simulink model "Motors_PID_Simulink_Cosimulation"  (R2019b)
settings: Solver=VariableStepAuto  StartTime=0.0  StopTime=10  FixedStep=0.0001  RelTol=1e-3
values from neighbouring files (symbols this model uses):
  desired_angle_vectors = deg2rad(desired_angles_deg)    [Motors_Main_Project.m]
  EKb = Kb(3)    [Motors_Main_Project.m]
  EKm = Km(3)    [Motors_Main_Project.m]
  EL = L(3)    [Motors_Main_Project.m]
  SKb = Kb(4)    [Motors_Main_Project.m]
  SKm = Km(4)    [Motors_Main_Project.m]
  SL = L(4)    [Motors_Main_Project.m]
  WKb = Kb(2)    [Motors_Main_Project.m]
  WKm = Km(2)    [Motors_Main_Project.m]
  WL = L(2)    [Motors_Main_Project.m]
undefined symbols (not defined in the file or in its folder): ER, GR, SR
libraries: cstblocks x4, simulink x4
settings Model: Creator=harsh  LastModifiedBy=harsh

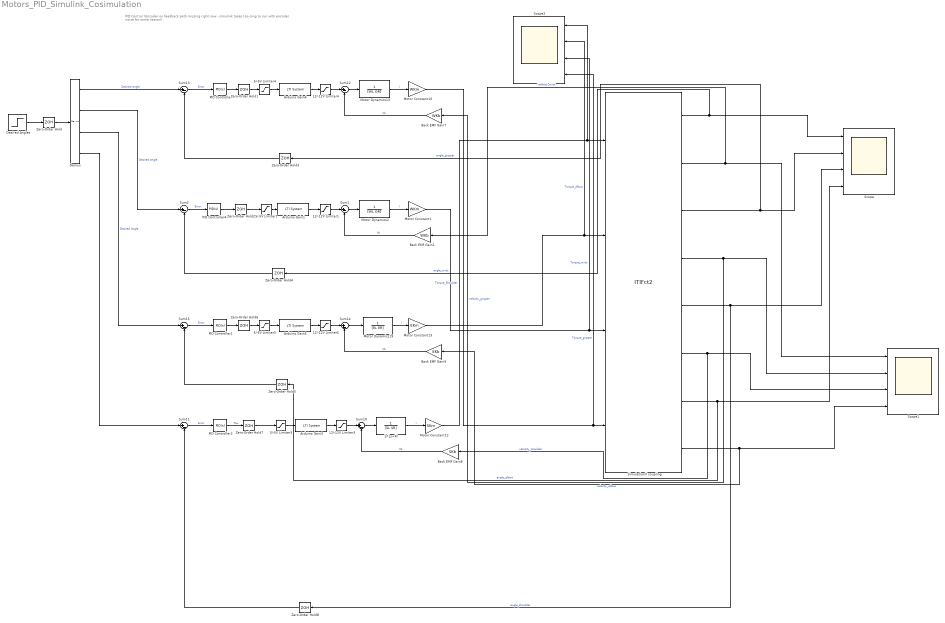
== system Motors_PID_Simulink_Cosimulation ==
  note: PID Control
      | (Encoder on feedback path missing right now - simulink takes too long to run with encoder noise for some reason)
  1/(Ls+R) : TransferFcn  Denominator=[SL SR]
  12/-12V Limiter{1,3..5} (4 alike) : Saturate  UpperLimit=12  LowerLimit=-12
  5/-5V Limiter{1,3..5} (4 alike) : Saturate  UpperLimit=5  LowerLimit=-5
  Arduino Gain1 : cstblocks/LTI System  sys=WOPAMP  IC=[]
  Arduino Gain3 : cstblocks/LTI System  sys=SOPAMP  IC=[]
  Arduino Gain4 : cstblocks/LTI System  sys=GOPAMP  IC=[]
  Arduino Gain5 : cstblocks/LTI System  sys=EOPAMP  IC=[]
  Back EMF Gain1 : Gain  Gain=WKb
  Back EMF Gain7 : Gain  Gain=WKb
  Back EMF Gain8 : Gain  Gain=SKb
  Back EMF Gain9 : Gain  Gain=EKb
  Demux : Demux
  "Desired Angles " : Step  Time=0.1  After=desired_angle_vectors  SampleTime=0
  Motor Constant1 : Gain  Gain=WKm
  Motor Constant10 : Gain  Gain=WKm
  Motor Constant12 : Gain  Gain=SKm
  Motor Constant13 : Gain  Gain=EKm
  Motor Dynamics13 : TransferFcn  Denominator=[WL GR]
  Motor Dynamics19 : TransferFcn  Denominator=[EL ER]
  Motor Dynamics2 : TransferFcn  Denominator=[WL GR]
  PID Controller : simulink/Continuous/PID Controller  Controller=PID  Form=Parallel  TimeDomain=Continuous-time  SampleTime=-1  IntegratorMethod=Forward Euler  FilterMethod=Forward Euler  ControllerParametersSource=internal  P=0.3697  I=0.00525  D=0.54744  UseFilter=on  N=5000  TunerSelectOption=Transfer Function Based (PID Tuner App)  InitialConditionSource=internal  InitialConditionForIntegrator=0  InitialConditionForFilter=0  DifferentiatorICPrevScaledInput=0  ExternalReset=none  TrackingMode=off  Kt=1  LimitOutput=off  UpperSaturationLimit=inf  LowerSaturationLimit=-inf  LinearizeAsGain=on  AntiWindupMode=none  Kb=1  POutMin=[]  POutMax=[]  IOutMin=[]  IOutMax=[]  DOutMin=[]  DOutMax=[]  NOutMin=[]  NOutMax=[]  SumOutMin=[]  SumOutMax=[]  SaturationOutMin=[]  SaturationOutMax=[]  PParamMin=[]  PParamMax=[]  IParamMin=[]  IParamMax=[]  DParamMin=[]  DParamMax=[]  NParamMin=[]  NParamMax=[]  KbParamMin=[]  KbParamMax=[]  KtParamMin=[]  KtParamMax=[]  KbOutMin=[]  KbOutMax=[]  KtOutMin=[]  KtOutMax=[]  IntegratorOutMin=[]  IntegratorOutMax=[]  FilterOutMin=[]  FilterOutMax=[]  SumI1OutMin=[]  SumI1OutMax=[]  SumI2OutMin=[]  SumI2OutMax=[]  SumI3OutMin=[]  SumI3OutMax=[]  SumI4OutMin=[]  SumI4OutMax=[]  SumDOutMin=[]  SumDOutMax=[]  DifferentiatorOutMin=[]  DifferentiatorOutMax=[]  FilterDiffOutCoefMin=[]  FilterDiffOutCoefMax=[]  ReciprocalOutMin=[]  ReciprocalOutMax=[]  SumDenOutMin=[]  SumDenOutMax=[]  SumNumOutMin=[]  SumNumOutMax=[]  DivideOutMin=[]  DivideOutMax=[]  IntegratorContinuousStateAttributes=''  IntegratorStateMustResolveToSignalObject=off  IntegratorRTWStateStorageClass=Auto  FilterContinuousStateAttributes=''  FilterStateMustResolveToSignalObject=off  FilterRTWStateStorageClass=Auto  ParallelPVariant=InternalParameters  IdealPVariant=Disabled  IVariant=InternalParameters  DVariant=InternalParameters  IntegratorVariant=Continuous  SatVariant=Disabled  AWVariant=Passthrough  PCopyVariant=Disabled  TRVariant=Disabled  FdbkBlocksVariant=Forward  IdealPFdbkVariant=Disabled  SatFdbkVariant=Disabled  DerivativeFilterVariant=ContFilter  NVariant=InternalParameters  NCopyVariant=Disabled  FilterICVariant=InternalICsFilter  IntegratorICVariant=InternalICs  ExternalResetVariant=Disabled  TRSumVariant=Passthrough  SumFdbkVariant=Disabled  SumVariant=Sum_PID
  PID Controller1 : simulink/Continuous/PID Controller  Controller=PID  Form=Parallel  TimeDomain=Continuous-time  SampleTime=-1  IntegratorMethod=Forward Euler  FilterMethod=Forward Euler  ControllerParametersSource=internal  P=0.03697  I=0.000525  D=3.84744  UseFilter=on  N=5000  TunerSelectOption=Transfer Function Based (PID Tuner App)  InitialConditionSource=internal  InitialConditionForIntegrator=0  InitialConditionForFilter=0  DifferentiatorICPrevScaledInput=0  ExternalReset=none  TrackingMode=off  Kt=1  LimitOutput=off  UpperSaturationLimit=inf  LowerSaturationLimit=-inf  LinearizeAsGain=on  AntiWindupMode=none  Kb=1  POutMin=[]  POutMax=[]  IOutMin=[]  IOutMax=[]  DOutMin=[]  DOutMax=[]  NOutMin=[]  NOutMax=[]  SumOutMin=[]  SumOutMax=[]  SaturationOutMin=[]  SaturationOutMax=[]  PParamMin=[]  PParamMax=[]  IParamMin=[]  IParamMax=[]  DParamMin=[]  DParamMax=[]  NParamMin=[]  NParamMax=[]  KbParamMin=[]  KbParamMax=[]  KtParamMin=[]  KtParamMax=[]  KbOutMin=[]  KbOutMax=[]  KtOutMin=[]  KtOutMax=[]  IntegratorOutMin=[]  IntegratorOutMax=[]  FilterOutMin=[]  FilterOutMax=[]  SumI1OutMin=[]  SumI1OutMax=[]  SumI2OutMin=[]  SumI2OutMax=[]  SumI3OutMin=[]  SumI3OutMax=[]  SumI4OutMin=[]  SumI4OutMax=[]  SumDOutMin=[]  SumDOutMax=[]  DifferentiatorOutMin=[]  DifferentiatorOutMax=[]  FilterDiffOutCoefMin=[]  FilterDiffOutCoefMax=[]  ReciprocalOutMin=[]  ReciprocalOutMax=[]  SumDenOutMin=[]  SumDenOutMax=[]  SumNumOutMin=[]  SumNumOutMax=[]  DivideOutMin=[]  DivideOutMax=[]  IntegratorContinuousStateAttributes=''  IntegratorStateMustResolveToSignalObject=off  IntegratorRTWStateStorageClass=Auto  FilterContinuousStateAttributes=''  FilterStateMustResolveToSignalObject=off  FilterRTWStateStorageClass=Auto  ParallelPVariant=InternalParameters  IdealPVariant=Disabled  IVariant=InternalParameters  DVariant=InternalParameters  IntegratorVariant=Continuous  SatVariant=Disabled  AWVariant=Passthrough  PCopyVariant=Disabled  TRVariant=Disabled  FdbkBlocksVariant=Forward  IdealPFdbkVariant=Disabled  SatFdbkVariant=Disabled  DerivativeFilterVariant=ContFilter  NVariant=InternalParameters  NCopyVariant=Disabled  FilterICVariant=InternalICsFilter  IntegratorICVariant=InternalICs  ExternalResetVariant=Disabled  TRSumVariant=Passthrough  SumFdbkVariant=Disabled  SumVariant=Sum_PID
  PID Controller2 : simulink/Continuous/PID Controller  Controller=PID  Form=Parallel  TimeDomain=Continuous-time  SampleTime=-1  IntegratorMethod=Forward Euler  FilterMethod=Forward Euler  ControllerParametersSource=internal  P=0.03697  I=0.00525  D=0.84744  UseFilter=on  N=5000  TunerSelectOption=Transfer Function Based (PID Tuner App)  InitialConditionSource=internal  InitialConditionForIntegrator=0  InitialConditionForFilter=0  DifferentiatorICPrevScaledInput=0  ExternalReset=none  TrackingMode=off  Kt=1  LimitOutput=off  UpperSaturationLimit=inf  LowerSaturationLimit=-inf  LinearizeAsGain=on  AntiWindupMode=none  Kb=1  POutMin=[]  POutMax=[]  IOutMin=[]  IOutMax=[]  DOutMin=[]  DOutMax=[]  NOutMin=[]  NOutMax=[]  SumOutMin=[]  SumOutMax=[]  SaturationOutMin=[]  SaturationOutMax=[]  PParamMin=[]  PParamMax=[]  IParamMin=[]  IParamMax=[]  DParamMin=[]  DParamMax=[]  NParamMin=[]  NParamMax=[]  KbParamMin=[]  KbParamMax=[]  KtParamMin=[]  KtParamMax=[]  KbOutMin=[]  KbOutMax=[]  KtOutMin=[]  KtOutMax=[]  IntegratorOutMin=[]  IntegratorOutMax=[]  FilterOutMin=[]  FilterOutMax=[]  SumI1OutMin=[]  SumI1OutMax=[]  SumI2OutMin=[]  SumI2OutMax=[]  SumI3OutMin=[]  SumI3OutMax=[]  SumI4OutMin=[]  SumI4OutMax=[]  SumDOutMin=[]  SumDOutMax=[]  DifferentiatorOutMin=[]  DifferentiatorOutMax=[]  FilterDiffOutCoefMin=[]  FilterDiffOutCoefMax=[]  ReciprocalOutMin=[]  ReciprocalOutMax=[]  SumDenOutMin=[]  SumDenOutMax=[]  SumNumOutMin=[]  SumNumOutMax=[]  DivideOutMin=[]  DivideOutMax=[]  IntegratorContinuousStateAttributes=''  IntegratorStateMustResolveToSignalObject=off  IntegratorRTWStateStorageClass=Auto  FilterContinuousStateAttributes=''  FilterStateMustResolveToSignalObject=off  FilterRTWStateStorageClass=Auto  ParallelPVariant=InternalParameters  IdealPVariant=Disabled  IVariant=InternalParameters  DVariant=InternalParameters  IntegratorVariant=Continuous  SatVariant=Disabled  AWVariant=Passthrough  PCopyVariant=Disabled  TRVariant=Disabled  FdbkBlocksVariant=Forward  IdealPFdbkVariant=Disabled  SatFdbkVariant=Disabled  DerivativeFilterVariant=ContFilter  NVariant=InternalParameters  NCopyVariant=Disabled  FilterICVariant=InternalICsFilter  IntegratorICVariant=InternalICs  ExternalResetVariant=Disabled  TRSumVariant=Passthrough  SumFdbkVariant=Disabled  SumVariant=Sum_PID
  PID Controller4 : simulink/Continuous/PID Controller  Controller=PID  Form=Parallel  TimeDomain=Continuous-time  SampleTime=-1  IntegratorMethod=Forward Euler  FilterMethod=Forward Euler  ControllerParametersSource=internal  P=0.3697  I=0.00525  D=0.74744  UseFilter=on  N=5000  TunerSelectOption=Transfer Function Based (PID Tuner App)  InitialConditionSource=internal  InitialConditionForIntegrator=0  InitialConditionForFilter=0  DifferentiatorICPrevScaledInput=0  ExternalReset=none  TrackingMode=off  Kt=1  LimitOutput=off  UpperSaturationLimit=inf  LowerSaturationLimit=-inf  LinearizeAsGain=on  AntiWindupMode=none  Kb=1  POutMin=[]  POutMax=[]  IOutMin=[]  IOutMax=[]  DOutMin=[]  DOutMax=[]  NOutMin=[]  NOutMax=[]  SumOutMin=[]  SumOutMax=[]  SaturationOutMin=[]  SaturationOutMax=[]  PParamMin=[]  PParamMax=[]  IParamMin=[]  IParamMax=[]  DParamMin=[]  DParamMax=[]  NParamMin=[]  NParamMax=[]  KbParamMin=[]  KbParamMax=[]  KtParamMin=[]  KtParamMax=[]  KbOutMin=[]  KbOutMax=[]  KtOutMin=[]  KtOutMax=[]  IntegratorOutMin=[]  IntegratorOutMax=[]  FilterOutMin=[]  FilterOutMax=[]  SumI1OutMin=[]  SumI1OutMax=[]  SumI2OutMin=[]  SumI2OutMax=[]  SumI3OutMin=[]  SumI3OutMax=[]  SumI4OutMin=[]  SumI4OutMax=[]  SumDOutMin=[]  SumDOutMax=[]  DifferentiatorOutMin=[]  DifferentiatorOutMax=[]  FilterDiffOutCoefMin=[]  FilterDiffOutCoefMax=[]  ReciprocalOutMin=[]  ReciprocalOutMax=[]  SumDenOutMin=[]  SumDenOutMax=[]  SumNumOutMin=[]  SumNumOutMax=[]  DivideOutMin=[]  DivideOutMax=[]  IntegratorContinuousStateAttributes=''  IntegratorStateMustResolveToSignalObject=off  IntegratorRTWStateStorageClass=Auto  FilterContinuousStateAttributes=''  FilterStateMustResolveToSignalObject=off  FilterRTWStateStorageClass=Auto  ParallelPVariant=InternalParameters  IdealPVariant=Disabled  IVariant=InternalParameters  DVariant=InternalParameters  IntegratorVariant=Continuous  SatVariant=Disabled  AWVariant=Passthrough  PCopyVariant=Disabled  TRVariant=Disabled  FdbkBlocksVariant=Forward  IdealPFdbkVariant=Disabled  SatFdbkVariant=Disabled  DerivativeFilterVariant=ContFilter  NVariant=InternalParameters  NCopyVariant=Disabled  FilterICVariant=InternalICsFilter  IntegratorICVariant=InternalICs  ExternalResetVariant=Disabled  TRSumVariant=Passthrough  SumFdbkVariant=Disabled  SumVariant=Sum_PID
  Scope : Scope  NumInputPorts=4
  Scope1 : Scope  NumInputPorts=4
  Scope2 : Scope  NumInputPorts=4
  SimulationX coupling : S-Function  FunctionName=ITIFct2  Parameters=ip, port, ts, nIn, nOut  SFunctionDeploymentMode=off  EnableBusSupport=off  mask{ip='localhost', port=1025, ts=0.005, nIn=4, nOut=8}
      mask prompts: ip "Address: ip"; port "Port Number: port [-]"; ts "Communication Step Size: ts [s]"; nIn "Input Vector Dimension (to SimulationX): nIn [-]"; nOut "Output Vector Dimension (from SimulationX): nOut [-]"
      mask help: Coupling Element
  Sum{1..2,10..15} (8 alike) : Sum  Inputs=|+-
  Zero-Order Hold{,1,3..8} (8 alike) : ZeroOrderHold  SampleTime=0.0001
  Zero-Order Hold2 : ZeroOrderHold  SampleTime=-1
  wires:
  "Desired Angles "/1 -> Zero-Order Hold/1
  5/-5V Limiter4/1 -> Arduino Gain4/1
  Arduino Gain4/1 -> 12/-12V Limiter4/1
  Back EMF Gain7/1 -> Sum12/2  "Vb"
  Sum12/1 -> Motor Dynamics13/1
  Demux/1 -> Sum13/1  "Desired angle"
  12/-12V Limiter4/1 -> Sum12/1
  Motor Dynamics13/1 -> Motor Constant10/1  "I"
  Motor Constant10/1 -> Scope2/4, SimulationX coupling/4  "Torque_gripper"
  Sum13/1 -> PID Controller/1  "Error"
  Sum2/1 -> PID Controller4/1  "Error"
  12/-12V Limiter1/1 -> Sum1/1
  Motor Dynamics2/1 -> Motor Constant1/1  "I"
  Sum1/1 -> Motor Dynamics2/1
  5/-5V Limiter1/1 -> Arduino Gain1/1
  Back EMF Gain1/1 -> Sum1/2  "Vb"
  Arduino Gain1/1 -> 12/-12V Limiter1/1
  Demux/2 -> Sum2/1  "Desired angle"
  PID Controller1/1 -> Zero-Order Hold6/1
  Sum15/1 -> PID Controller1/1  "Error"
  Motor Dynamics19/1 -> Motor Constant13/1  "I"
  Motor Constant13/1 -> Scope2/2, SimulationX coupling/2  "Torque_elbow"
  12/-12V Limiter5/1 -> Sum14/1
  Sum14/1 -> Motor Dynamics19/1
  5/-5V Limiter5/1 -> Arduino Gain5/1
  Back EMF Gain9/1 -> Sum14/2  "Vb"
  Arduino Gain5/1 -> 12/-12V Limiter5/1
  Demux/3 -> Sum15/1  "Desired Angle"
  Back EMF Gain8/1 -> Sum10/2  "Vb"
  Motor Constant12/1 -> SimulationX coupling/1, Scope2/1  "Torque_Shoulder"
  5/-5V Limiter3/1 -> Arduino Gain3/1
  Arduino Gain3/1 -> 12/-12V Limiter3/1
  1/(Ls+R)/1 -> Motor Constant12/1  "I"
  12/-12V Limiter3/1 -> Sum10/1
  PID Controller2/1 -> Zero-Order Hold7/1  "Tau"
  Sum11/1 -> PID Controller2/1  "Error"
  Sum10/1 -> 1/(Ls+R)/1
  Demux/4 -> Sum11/1
  PID Controller4/1 -> Zero-Order Hold2/1
  PID Controller/1 -> Zero-Order Hold1/1
  Zero-Order Hold/1 -> Demux/1
  Zero-Order Hold1/1 -> 5/-5V Limiter4/1
  Zero-Order Hold2/1 -> 5/-5V Limiter1/1
  Zero-Order Hold3/1 -> Sum13/2
  Zero-Order Hold4/1 -> Sum2/2
  Zero-Order Hold5/1 -> Sum15/2
  Zero-Order Hold6/1 -> 5/-5V Limiter5/1
  Zero-Order Hold7/1 -> 5/-5V Limiter3/1
  Zero-Order Hold8/1 -> Sum11/2
  SimulationX coupling/2 -> Back EMF Gain1/1, Scope1/1  "velocity_wrist"
  SimulationX coupling/1 -> Zero-Order Hold4/1, Scope/1  "angle_wrist"
  SimulationX coupling/3 -> Zero-Order Hold3/1, Scope/2  "angle_gripper"
  SimulationX coupling/4 -> Back EMF Gain7/1, Scope1/2  "velocity_gripper"
  Motor Constant1/1 -> Scope2/3, SimulationX coupling/3  "Torque_wrist"
  SimulationX coupling/5 -> Zero-Order Hold8/1, Scope/3  "angle_shoulder"
  SimulationX coupling/6 -> Back EMF Gain8/1, Scope1/3  "velocity_shoulder"
  SimulationX coupling/7 -> Zero-Order Hold5/1, Scope/4  "angle_elbow"
  SimulationX coupling/8 -> Back EMF Gain9/1, Scope1/4  "velocity_elbow"
